simulink model "P2d_PI"  (R2014a)
settings: Solver=ode45  StartTime=0.0  StopTime=1200  RelTol=1e-3
undefined symbols (not defined in the file): beta, c1, c2, idss, modelo_lineal_rango_alto, modelo_lineal_rango_bajo, modelo_lineal_rango_medio
libraries: simulink x3, slident x3
settings Model: Creator=matias  LastModifiedBy=pdoren
settings DataIOCC: SignalLoggingSaveFormat=ModelDataLogs
settings OptimizationCC: ExpressionDepthLimit=2147483647
settings DebuggingCC: UnderspecifiedInitializationDetection=Classic  FcnCallInpInsideContextMsg=EnableAllAsWarning  StateNameClashWarn=warning

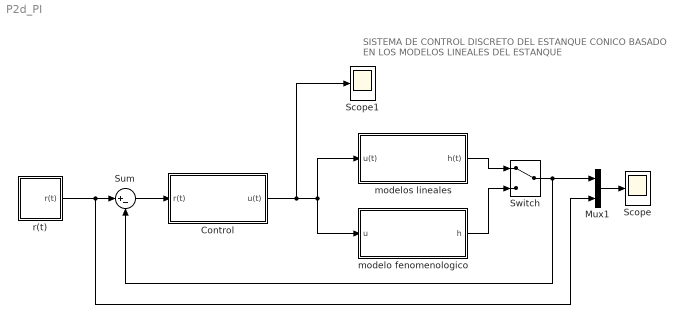
== system P2d_PI ==
  note: SISTEMA DE CONTROL DISCRETO DEL ESTANQUE CONICO
      | BASADO EN LOS MODELOS LINEALES DEL ESTANQUE
  Control : Subsystem
  Mux1 : Mux  Inputs=2
  Scope : Scope
      settings: TimeRange=1200  YMin=22.6  YMax=25
  Scope1 : Scope
  Sum : Sum  Inputs=|+-
  Switch : ManualSwitch
  modelo fenomenologico : Subsystem  Tag=Modelo Fenomenologico
  modelos lineales : Subsystem  Tag=Modelo Fenomenologico
  r(t) : Subsystem
  wires:
  Mux1/1 -> Scope/1
  r(t)/1(r(t)) -> Mux1/2, Sum/1
  Control/1(u(t)) -> Scope1/1, modelo fenomenologico/1(u), modelos lineales/1(u(t))
  Sum/1 -> Control/1(r(t))
  Switch/1 -> Sum/2, Mux1/1
  modelos lineales/1(h(t)) -> Switch/1
  modelo fenomenologico/1(h) -> Switch/2

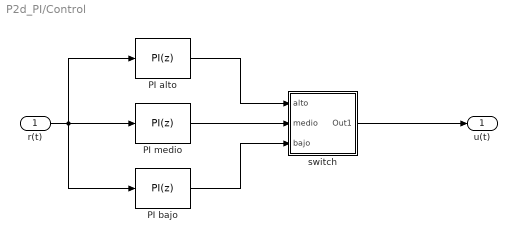
== system P2d_PI/Control ==
  r(t) : Inport
  PI alto : simulink/Continuous/PID Controller  Controller=PI  TimeDomain=Discrete-time  SampleTime=0.5  IntegratorMethod=Forward Euler  FilterMethod=Forward Euler  Form=Parallel  P=54  I=(1-0.995)*54*0.1/0.5  D=0  N=100  InitialConditionSource=internal  InitialConditionForIntegrator=0  InitialConditionForFilter=0  ExternalReset=none  LimitOutput=on  UpperSaturationLimit=100  LowerSaturationLimit=0  LinearizeAsGain=off  AntiWindupMode=none  Kb=1  TrackingMode=off  Kt=1  PParamMin=[]  PParamMax=[]  IParamMin=[]  IParamMax=[]  DParamMin=[]  DParamMax=[]  NParamMin=[]  NParamMax=[]  KbParamMin=[]  KbParamMax=[]  KtParamMin=[]  KtParamMax=[]  POutMin=[]  POutMax=[]  IOutMin=[]  IOutMax=[]  DOutMin=[]  DOutMax=[]  NOutMin=[]  NOutMax=[]  KbOutMin=[]  KbOutMax=[]  KtOutMin=[]  KtOutMax=[]  IntegratorOutMin=[]  IntegratorOutMax=[]  FilterOutMin=[]  FilterOutMax=[]  SumOutMin=[]  SumOutMax=[]  SumI1OutMin=[]  SumI1OutMax=[]  SumI2OutMin=[]  SumI2OutMax=[]  SumI3OutMin=[]  SumI3OutMax=[]  SumDOutMin=[]  SumDOutMax=[]  SaturationOutMin=[]  SaturationOutMax=[]  IntegratorContinuousStateAttributes=''  IntegratorStateMustResolveToSignalObject=off  IntegratorRTWStateStorageClass=Auto  FilterContinuousStateAttributes=''  FilterStateMustResolveToSignalObject=off  FilterRTWStateStorageClass=Auto
  PI bajo : simulink/Continuous/PID Controller  Controller=PI  TimeDomain=Discrete-time  SampleTime=0.5  IntegratorMethod=Forward Euler  FilterMethod=Forward Euler  Form=Parallel  P=46  I=(1-0.952)*46*0.1/0.5  D=0  N=100  InitialConditionSource=internal  InitialConditionForIntegrator=0  InitialConditionForFilter=0  ExternalReset=none  LimitOutput=on  UpperSaturationLimit=100  LowerSaturationLimit=0  LinearizeAsGain=off  AntiWindupMode=none  Kb=1  TrackingMode=off  Kt=1  PParamMin=[]  PParamMax=[]  IParamMin=[]  IParamMax=[]  DParamMin=[]  DParamMax=[]  NParamMin=[]  NParamMax=[]  KbParamMin=[]  KbParamMax=[]  KtParamMin=[]  KtParamMax=[]  POutMin=[]  POutMax=[]  IOutMin=[]  IOutMax=[]  DOutMin=[]  DOutMax=[]  NOutMin=[]  NOutMax=[]  KbOutMin=[]  KbOutMax=[]  KtOutMin=[]  KtOutMax=[]  IntegratorOutMin=[]  IntegratorOutMax=[]  FilterOutMin=[]  FilterOutMax=[]  SumOutMin=[]  SumOutMax=[]  SumI1OutMin=[]  SumI1OutMax=[]  SumI2OutMin=[]  SumI2OutMax=[]  SumI3OutMin=[]  SumI3OutMax=[]  SumDOutMin=[]  SumDOutMax=[]  SaturationOutMin=[]  SaturationOutMax=[]  IntegratorContinuousStateAttributes=''  IntegratorStateMustResolveToSignalObject=off  IntegratorRTWStateStorageClass=Auto  FilterContinuousStateAttributes=''  FilterStateMustResolveToSignalObject=off  FilterRTWStateStorageClass=Auto
  PI medio : simulink/Continuous/PID Controller  Controller=PI  TimeDomain=Discrete-time  SampleTime=0.5  IntegratorMethod=Forward Euler  FilterMethod=Forward Euler  Form=Parallel  P=50  I=(1-0.995)*50*0.3/0.5  D=0  N=100  InitialConditionSource=internal  InitialConditionForIntegrator=0  InitialConditionForFilter=0  ExternalReset=none  LimitOutput=on  UpperSaturationLimit=100  LowerSaturationLimit=0  LinearizeAsGain=off  AntiWindupMode=none  Kb=1  TrackingMode=off  Kt=1  PParamMin=[]  PParamMax=[]  IParamMin=[]  IParamMax=[]  DParamMin=[]  DParamMax=[]  NParamMin=[]  NParamMax=[]  KbParamMin=[]  KbParamMax=[]  KtParamMin=[]  KtParamMax=[]  POutMin=[]  POutMax=[]  IOutMin=[]  IOutMax=[]  DOutMin=[]  DOutMax=[]  NOutMin=[]  NOutMax=[]  KbOutMin=[]  KbOutMax=[]  KtOutMin=[]  KtOutMax=[]  IntegratorOutMin=[]  IntegratorOutMax=[]  FilterOutMin=[]  FilterOutMax=[]  SumOutMin=[]  SumOutMax=[]  SumI1OutMin=[]  SumI1OutMax=[]  SumI2OutMin=[]  SumI2OutMax=[]  SumI3OutMin=[]  SumI3OutMax=[]  SumDOutMin=[]  SumDOutMax=[]  SaturationOutMin=[]  SaturationOutMax=[]  IntegratorContinuousStateAttributes=''  IntegratorStateMustResolveToSignalObject=off  IntegratorRTWStateStorageClass=Auto  FilterContinuousStateAttributes=''  FilterStateMustResolveToSignalObject=off  FilterRTWStateStorageClass=Auto
  switch : Subsystem
  u(t) : Outport
  wires:
  r(t)/1 -> PI bajo/1, PI medio/1, PI alto/1
  switch/1(Out1) -> u(t)/1
  PI alto/1 -> switch/1(alto)
  PI medio/1 -> switch/2(medio)
  PI bajo/1 -> switch/3(bajo)

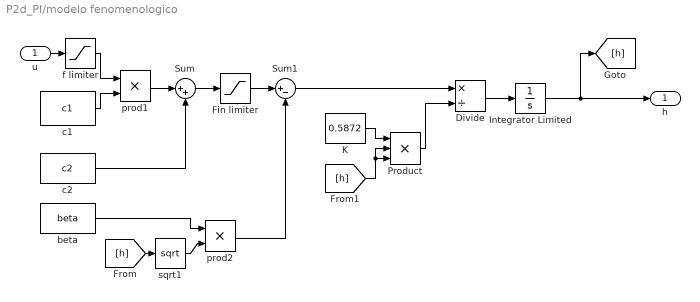
== system P2d_PI/modelo fenomenologico ==
  u : Inport
  Divide : Product  Inputs=*/
  Fin limiter : Saturate  UpperLimit=inf  LowerLimit=0
  Integrator Limited : Integrator  InitialCondition=0.1  LimitOutput=on  UpperSaturationLimit=80  LowerSaturationLimit=0.1
  K : Constant  Value=0.5872
  Product : Product  Inputs=3  RndMeth=Zero
  Sum : Sum  Inputs=|++
  Sum1 : Sum  Inputs=|+-
  beta : Constant  Value=beta
  c1 : Constant  Value=c1
  c2 : Constant  Value=c2
  f limiter : Saturate  UpperLimit=100  LowerLimit=0
  prod1 : Product  RndMeth=Zero
  prod2 : Product  RndMeth=Zero
  sqrt1 : Sqrt  SaturateOnIntegerOverflow=on
  h : Outport
  wires:
  f limiter/1 -> prod1/1
  c1/1 -> prod1/2
  prod1/1 -> Sum/1
  c2/1 -> Sum/2
  beta/1 -> prod2/1
  prod2/1 -> Sum1/2
  sqrt1/1 -> prod2/2
  Sum1/1 -> Divide/1
  [h] -> sqrt1/1
  Product/1 -> Divide/2
  K/1 -> Product/1
  [h] -> Product/2, Product/3
  Divide/1 -> Integrator Limited/1
  Integrator Limited/1 -> h/1, [h]
  Sum/1 -> Fin limiter/1
  Fin limiter/1 -> Sum1/1
  u/1 -> f limiter/1

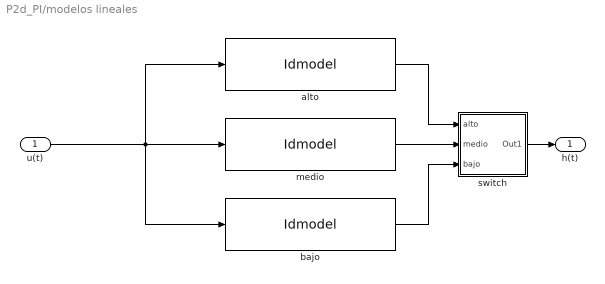
== system P2d_PI/modelos lineales ==
  u(t) : Inport
  alto : slident/Models/Idmodel  sys=idss(modelo_lineal_rango_alto)  IC=X0_alto  noi=on  seed=[]
  bajo : slident/Models/Idmodel  sys=idss(modelo_lineal_rango_bajo)  IC=X0_bajo  noi=on  seed=[]
  medio : slident/Models/Idmodel  sys=idss(modelo_lineal_rango_medio)  IC=X0_medio  noi=on  seed=[]
  switch : Subsystem
  h(t) : Outport
  wires:
  u(t)/1 -> bajo/1, alto/1, medio/1
  medio/1 -> switch/2(medio)
  switch/1(Out1) -> h(t)/1
  bajo/1 -> switch/3(bajo)
  alto/1 -> switch/1(alto)

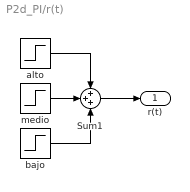
== system P2d_PI/r(t) ==
  Sum1 : Sum  Inputs=+++
  alto : Step  Time=800  After=15  SampleTime=0
  bajo : Step  Time=0  After=25  SampleTime=0
  medio : Step  Time=400  After=15  SampleTime=0
  r(t) : Outport
  wires:
  alto/1 -> Sum1/1
  bajo/1 -> Sum1/3
  Sum1/1 -> r(t)/1
  medio/1 -> Sum1/2

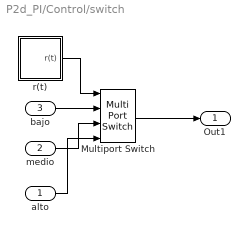
== system P2d_PI/Control/switch ==
  alto : Inport
  medio : Inport  Port=2
  bajo : Inport  Port=3
  Multiport Switch : MultiPortSwitch
  r(t) : Subsystem
  Out1 : Outport
  wires:
  Multiport Switch/1 -> Out1/1
  bajo/1 -> Multiport Switch/2
  medio/1 -> Multiport Switch/3
  alto/1 -> Multiport Switch/4
  r(t)/1(r(t)) -> Multiport Switch/1

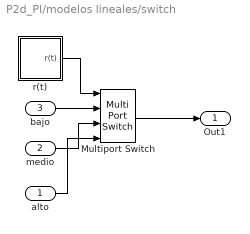
== system P2d_PI/modelos lineales/switch ==
  alto : Inport
  medio : Inport  Port=2
  bajo : Inport  Port=3
  Multiport Switch : MultiPortSwitch
  r(t) : Subsystem
  Out1 : Outport
  wires:
  Multiport Switch/1 -> Out1/1
  bajo/1 -> Multiport Switch/2
  medio/1 -> Multiport Switch/3
  alto/1 -> Multiport Switch/4
  r(t)/1(r(t)) -> Multiport Switch/1

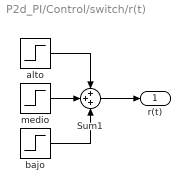
== system P2d_PI/Control/switch/r(t) ==
  Sum1 : Sum  Inputs=+++
  alto : Step  Time=800  SampleTime=0
  bajo : Step  Time=0  SampleTime=0
  medio : Step  Time=400  SampleTime=0
  r(t) : Outport
  wires:
  alto/1 -> Sum1/1
  bajo/1 -> Sum1/3
  Sum1/1 -> r(t)/1
  medio/1 -> Sum1/2

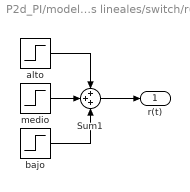
== system P2d_PI/modelos lineales/switch/r(t) ==
  Sum1 : Sum  Inputs=+++
  alto : Step  Time=800  SampleTime=0
  bajo : Step  Time=0  SampleTime=0
  medio : Step  Time=400  SampleTime=0
  r(t) : Outport
  wires:
  alto/1 -> Sum1/1
  bajo/1 -> Sum1/3
  Sum1/1 -> r(t)/1
  medio/1 -> Sum1/2
